simulink model "CONTROLLER_LONG_FG"  (R2015a)
settings: Solver=ode45  StartTime=0.0  StopTime=196  RelTol=1e-3
values from neighbouring files (symbols this model uses):
  A = [-0.0089 -0.1474 0 -9.75; -0.0216 -0.3601 5.9470 -0.151; 0 -0.00015 -0.0224 0.0006; 0 0 1 0]    [controller_design.m]
  B = [-2.682 9.748; 29 3.77; -3.847 -0.034; 0 0]    [controller_design.m]
  C = diag([1 1 1 1])    [controller_design.m]
  D = zeros(4,2)    [controller_design.m]
  K = place(A,B,p)    [controller_design.m]
  tht_tr = 6.30*(pi/180)    (= 0.109955742876)    [controller_design.m]
  u_tr = 155    [controller_design.m]
  w_tr = 0    [controller_design.m]
  XE_0 = 0    [constants.m]    (also in controller_design.m)
  ZE_0 = -2000    [constants.m]    (also in controller_design.m)
undefined symbols (not defined in the file or in its folder): Earth, magnitude, WGS84
libraries: simulink x3, aerolibtransform2 x2, aerolibfltsims x1
settings Model: Creator=vinay  LastModifiedBy=vinay

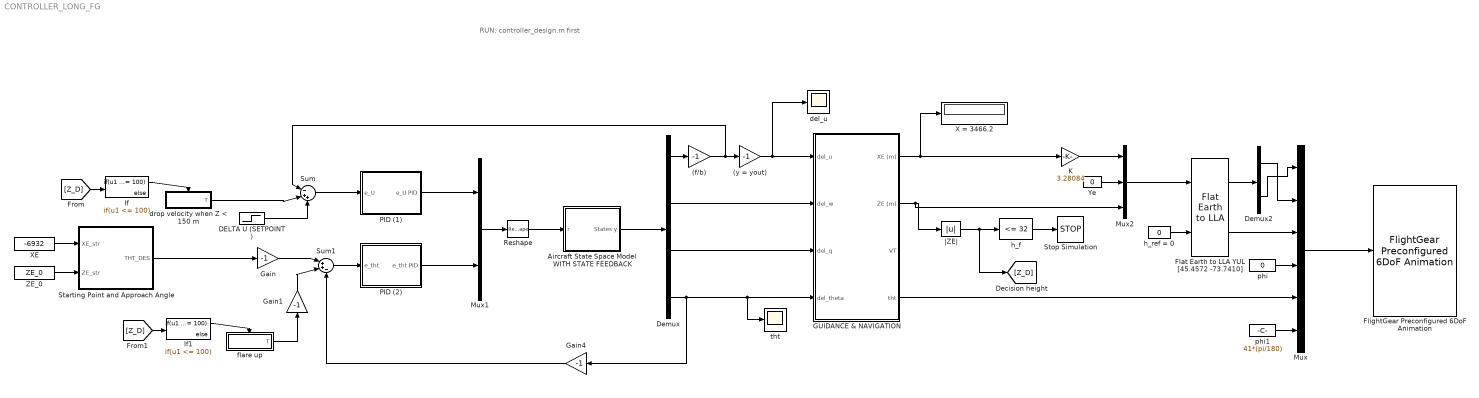
== system CONTROLLER_LONG_FG ==
  note: RUN: controller_design.m first
  (f/b) : Gain  Gain=-1
  (y = yout) : Gain  Gain=-1
  Aircraft State Space Model WITH STATE FEEDBACK : Subsystem
  DELTA U (SETPOINT) : Step  After=36  SampleTime=0
  Demux : Demux
  Demux2 : Demux  Outputs=2
  "Flat Earth to LLA YUL [45.4572 -73.7410] " : aerolibtransform2/Flat Earth to LLA  units=Metric (MKS)  ptype=Earth (WGS84)  F=1/298.257223563  R=6378137  LL0=[45.3027633 -73.9311585]  psi=41
  FlightGear Preconfigured 6DoF Animation : aerolibfltsims/FlightGear Preconfigured 6DoF Animation  xFlightGearVersion=v3.0  DestinationIpAddress=127.0.0.1  DestinationPort=5502  SampleTime=1/30
  "GUIDANCE & NAVIGATION " : Subsystem
  Gain : Gain  Gain=-1
  Gain1 : Gain  Gain=-1
  Gain4 : Gain  Gain=-1
  If : If  IfExpression=u1 <= 100
  If1 : If  IfExpression=u1 <= 100
  K : Gain  Gain=3.28084
  Mux : Mux  Inputs=6
  Mux1 : Mux  Inputs=2
  Mux2 : Mux  Inputs=3
  PID (1) : Subsystem
  PID (2) : Subsystem
  Reshape : Reshape  OutputDimensionality=Customize  OutputDimensions=[2,1]
  Starting Point and Approach Angle : Subsystem
  Stop Simulation : Stop
  Sum : Sum  Inputs=|-++
  Sum1 : Sum  Inputs=|++-
  X = 3466.2 : Display
  "XE " : Constant  Value=-6932
  Ye : Constant  Value=0
  ZE_0 : Constant  Value=ZE_0
  del_u : Scope
      settings: YMin=-1.225e+06  YMax=-800000
  drop velocity when Z < 150 m : Subsystem  TreatAsAtomicUnit=on
  flare up : Subsystem  TreatAsAtomicUnit=on
  h_f : simulink/Logic and Bit Operations/Compare To Constant  relop=<=  const=32  OutDataTypeStr=boolean
  h_ref = 0 : Constant  Value=0
  phi : Constant  Value=0
  phi1 : Constant  Value=41*(pi/180)
  tht : Scope
      settings: YMin=-57500  YMax=-10000
  |ZE| : Abs
  wires:
  Mux1/1 -> Reshape/1
  Reshape/1 -> Aircraft State Space Model WITH STATE FEEDBACK/1(r)
  Aircraft State Space Model WITH STATE FEEDBACK/1(States y) -> Demux/1
  ? -> ?
  Demux/1 -> (f/b)/1
  Gain/1 -> Sum1/1
  Demux/4 -> "GUIDANCE & NAVIGATION "/4(del_theta), tht/1, Gain4/1
  Sum/1 -> PID (1)/1(e_U)
  PID (1)/1(e_U PID) -> Mux1/1
  Sum1/1 -> PID (2)/1(e_tht)
  PID (2)/1(e_tht PID) -> Mux1/2
  Demux/2 -> "GUIDANCE & NAVIGATION "/2(del_w)
  Demux/3 -> "GUIDANCE & NAVIGATION "/3(del_q)
  "GUIDANCE & NAVIGATION "/2(ZE (m)) -> Mux2/3, |ZE|/1
  |ZE|/1 -> [Z_D], h_f/1
  "XE "/1 -> Starting Point and Approach Angle/1(XE_str)
  ZE_0/1 -> Starting Point and Approach Angle/2(ZE_str)
  Starting Point and Approach Angle/1(THT_DES) -> Gain/1
  h_f/1 -> Stop Simulation/1
  (y = yout)/1 -> del_u/1, "GUIDANCE & NAVIGATION "/1(del_u)
  Mux/1 -> FlightGear Preconfigured 6DoF Animation/1
  phi/1 -> Mux/4
  phi1/1 -> Mux/6
  "GUIDANCE & NAVIGATION "/1(XE (m)) -> X = 3466.2/1, K/1
  Ye/1 -> Mux2/2
  Mux2/1 -> "Flat Earth to LLA YUL [45.4572 -73.7410] "/1
  h_ref = 0/1 -> "Flat Earth to LLA YUL [45.4572 -73.7410] "/2
  "Flat Earth to LLA YUL [45.4572 -73.7410] "/1 -> Demux2/1
  "Flat Earth to LLA YUL [45.4572 -73.7410] "/2 -> Mux/3
  Demux2/1 -> Mux/2
  Demux2/2 -> Mux/1
  "GUIDANCE & NAVIGATION "/4(tht) -> Mux/5
  K/1 -> Mux2/1
  DELTA U (SETPOINT)/1 -> Sum/3
  If/1 -> drop velocity when Z < 150 m/Action
  [Z_D] -> If/1
  Gain4/1 -> Sum1/3
  If1/1 -> flare up/Action
  [Z_D] -> If1/1
  drop velocity when Z < 150 m/1(T) -> Sum/2
  (f/b)/1 -> Sum/1, (y = yout)/1
  flare up/1(T) -> Gain1/1
  Gain1/1 -> Sum1/2

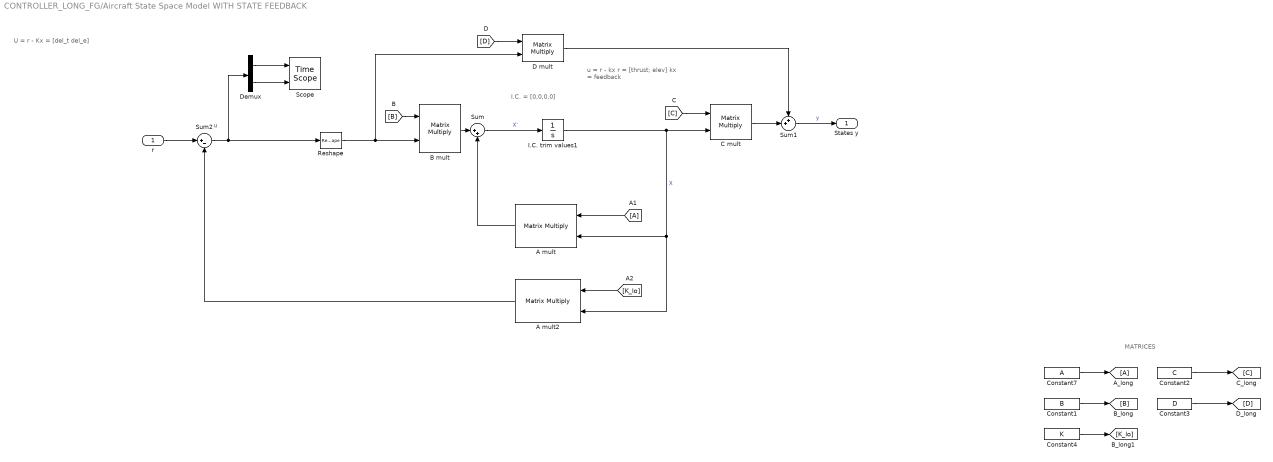
== system CONTROLLER_LONG_FG/Aircraft State Space Model WITH STATE FEEDBACK ==
  note: u
  note: U = r - Kx = [del_t del_e]
  note: u = r - kx
      | r = [thrust; elev]
      | kx = feedback
  note: MATRICES
  note: I.C. = [0,0,0,0]
  r : Inport
  A mult : Product  Multiplication=Matrix(*)  RndMeth=Zero
  A mult2 : Product  Multiplication=Matrix(*)  RndMeth=Zero
  B mult : Product  Multiplication=Matrix(*)  RndMeth=Zero
  C mult : Product  Multiplication=Matrix(*)  RndMeth=Zero
  Constant1 : Constant  Value=B
  Constant2 : Constant  Value=C
  Constant3 : Constant  Value=D
  Constant4 : Constant  Value=K
  Constant7 : Constant  Value=A
  D mult : Product  Multiplication=Matrix(*)  RndMeth=Zero
  Demux : Demux  Outputs=2
  I.C. trim values1 : Integrator  InitialCondition=[0;0;0;0]
  Reshape : Reshape  OutputDimensionality=Customize  OutputDimensions=[2,1]
  Scope : TimeScope  NumInputPorts=2
  Sum : Sum  Inputs=|++
  Sum1 : Sum  Inputs=++|
  Sum2 : Sum  Inputs=|+-
  States y : Outport
  wires:
  Sum/1 -> I.C. trim values1/1  "X'"
  D mult/1 -> Sum1/1
  A mult/1 -> Sum/2
  [B] -> B mult/1
  [A] -> A mult/1
  [D] -> D mult/1
  [C] -> C mult/1
  Sum1/1 -> States y/1  "y"
  B mult/1 -> Sum/1
  C mult/1 -> Sum1/2
  Constant7/1 -> [A]
  Constant1/1 -> [B]
  Constant2/1 -> [C]
  Constant3/1 -> [D]
  Constant4/1 -> [K_lo]
  [K_lo] -> A mult2/1
  A mult2/1 -> Sum2/2
  r/1 -> Sum2/1
  Reshape/1 -> D mult/2, B mult/2
  I.C. trim values1/1 -> C mult/2, A mult2/2, A mult/2  "X"
  Sum2/1 -> Demux/1, Reshape/1
  Demux/1 -> Scope/1
  Demux/2 -> Scope/2

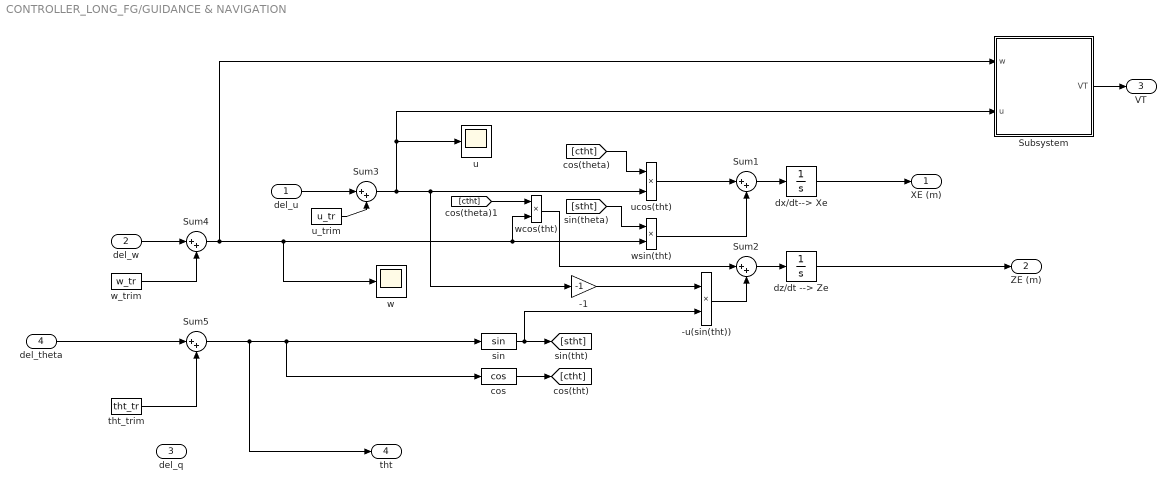
== system CONTROLLER_LONG_FG/GUIDANCE & NAVIGATION  ==
  del_u : Inport
  del_w : Inport  Port=2
  del_q : Inport  Port=3
  del_theta : Inport  Port=4
  -1 : Gain  Gain=-1
  -u(sin(tht)) : Product
  Subsystem : Subsystem
  Sum{1..5} (5 alike) : Sum  Inputs=|++
  cos : Trigonometry  Operator=cos
  dx/dt--> Xe : Integrator  InitialCondition=XE_0
  dz/dt --> Ze : Integrator  InitialCondition=ZE_0
  sin : Trigonometry
  tht_trim : Constant  Value=tht_tr
  u : Scope
      settings: SaveName=ScopeData4
  u_trim : Constant  Value=u_tr
  ucos(tht) : Product
  w : Scope
      settings: SaveName=ScopeData5
  w_trim : Constant  Value=w_tr
  wcos(tht) : Product
  wsin(tht) : Product
  XE (m) : Outport
  ZE (m) : Outport  Port=2
  VT : Outport  Port=3
  tht : Outport  Port=4
  wires:
  [stht] -> wsin(tht)/1
  wsin(tht)/1 -> Sum1/2
  dx/dt--> Xe/1 -> XE (m)/1
  ucos(tht)/1 -> Sum1/1
  dz/dt --> Ze/1 -> ZE (m)/1
  Sum1/1 -> dx/dt--> Xe/1
  Sum2/1 -> dz/dt --> Ze/1
  cos/1 -> [ctht]
  sin/1 -> -u(sin(tht))/2, [stht]
  wcos(tht)/1 -> Sum2/1
  [ctht] -> wcos(tht)/1
  -1/1 -> -u(sin(tht))/1
  [ctht] -> ucos(tht)/1
  -u(sin(tht))/1 -> Sum2/2
  tht_trim/1 -> Sum5/2
  del_u/1 -> Sum3/1
  Sum3/1 -> u/1, Subsystem/2(u), -1/1, ucos(tht)/2
  u_trim/1 -> Sum3/2
  del_w/1 -> Sum4/1
  Sum4/1 -> w/1, wcos(tht)/2, wsin(tht)/2, Subsystem/1(w)
  w_trim/1 -> Sum4/2
  del_theta/1 -> Sum5/1
  Sum5/1 -> tht/1, cos/1, sin/1
  Subsystem/1(VT) -> VT/1

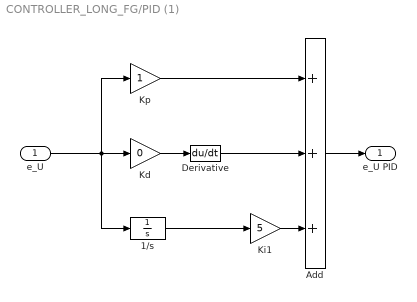
== system CONTROLLER_LONG_FG/PID (1) ==
  e_U : Inport
  1/s : Integrator
  Add : Sum  Inputs=+++
  Derivative : Derivative
  Kd : Gain  Gain=0
  Ki1 : Gain  Gain=5
  Kp : Gain
  e_U PID : Outport
  wires:
  Add/1 -> e_U PID/1
  Kp/1 -> Add/1
  Ki1/1 -> Add/3
  e_U/1 -> 1/s/1, Kd/1, Kp/1
  Kd/1 -> Derivative/1
  Derivative/1 -> Add/2
  1/s/1 -> Ki1/1

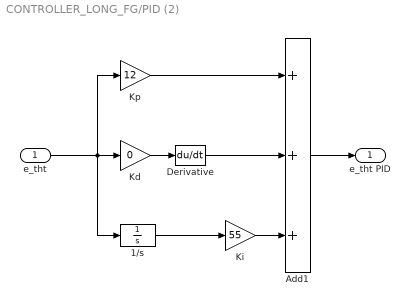
== system CONTROLLER_LONG_FG/PID (2) ==
  e_tht : Inport
  1/s : Integrator
  Add1 : Sum  Inputs=+++
  Derivative : Derivative
  "Kd " : Gain  Gain=0
  "Ki " : Gain  Gain=55
  Kp : Gain  Gain=12
  e_tht PID : Outport
  wires:
  Add1/1 -> e_tht PID/1
  Kp/1 -> Add1/1
  e_tht/1 -> Kp/1, 1/s/1, "Kd "/1
  "Ki "/1 -> Add1/3
  "Kd "/1 -> Derivative/1
  Derivative/1 -> Add1/2
  1/s/1 -> "Ki "/1

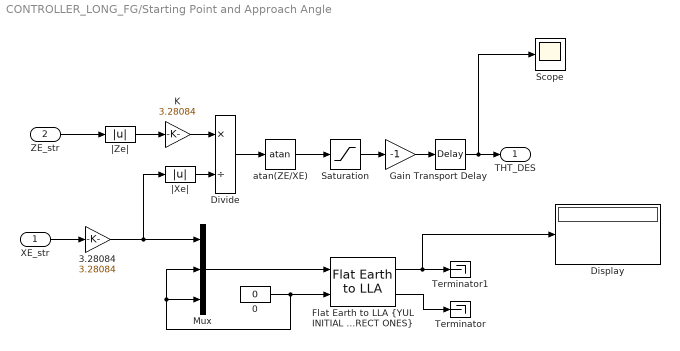
== system CONTROLLER_LONG_FG/Starting Point and Approach Angle ==
  XE_str : Inport
  ZE_str : Inport  Port=2
  0 : Constant  Value=0
  3.28084 : Gain  Gain=3.28084
  Display : Display
  Divide : Product  Inputs=*/
  "Flat Earth to LLA {YUL INITIAL COORDS UPDATED - CORRECT ONES}" : aerolibtransform2/Flat Earth to LLA  units=Metric (MKS)  ptype=Earth (WGS84)  F=1/298.257223563  R=6378137  LL0=[45.4572 -73.7410]  psi=41
  Gain : Gain  Gain=-1
  K : Gain  Gain=3.28084
  Mux : Mux  Inputs=3
  Saturation : Saturate  UpperLimit=0.5235  LowerLimit=-0.5235
  Scope : Scope
      settings: SaveName=ScopeData2
  Terminator : Terminator
  Terminator1 : Terminator
  Transport Delay : TransportDelay
  atan(ZE/XE) : Trigonometry  Operator=atan
  |Xe| : Abs
  |Ze| : Abs
  THT_DES : Outport
  wires:
  Mux/1 -> "Flat Earth to LLA {YUL INITIAL COORDS UPDATED - CORRECT ONES}"/1
  XE_str/1 -> 3.28084/1
  0/1 -> Mux/2, Mux/3, "Flat Earth to LLA {YUL INITIAL COORDS UPDATED - CORRECT ONES}"/2
  ZE_str/1 -> |Ze|/1
  |Ze|/1 -> K/1
  |Xe|/1 -> Divide/2
  Divide/1 -> atan(ZE/XE)/1
  "Flat Earth to LLA {YUL INITIAL COORDS UPDATED - CORRECT ONES}"/2 -> Terminator/1
  Saturation/1 -> Gain/1
  atan(ZE/XE)/1 -> Saturation/1
  Gain/1 -> Transport Delay/1
  Transport Delay/1 -> Scope/1, THT_DES/1
  "Flat Earth to LLA {YUL INITIAL COORDS UPDATED - CORRECT ONES}"/1 -> Display/1, Terminator1/1
  3.28084/1 -> |Xe|/1, Mux/1
  K/1 -> Divide/1

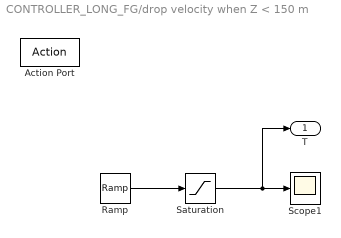
== system CONTROLLER_LONG_FG/drop velocity when Z < 150 m ==
  Action Port : ActionPort  ActionType=then
  Ramp : simulink/Sources/Ramp  slope=5  start=0  X0=0
  Saturation : Saturate  UpperLimit=15  LowerLimit=0
  Scope1 : Scope
      settings: TimeRange=11  YMin=0  YMax=3.5  SaveName=ScopeData2
  T : Outport
  wires:
  Ramp/1 -> Saturation/1
  Saturation/1 -> T/1, Scope1/1

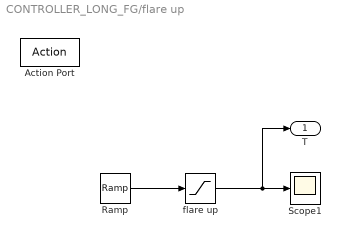
== system CONTROLLER_LONG_FG/flare up ==
  Action Port : ActionPort  ActionType=then
  Ramp : simulink/Sources/Ramp  slope=0.35  start=0  X0=0
  Scope1 : Scope
      settings: TimeRange=11  YMin=0  YMax=3.5  SaveName=ScopeData2
  flare up : Saturate  UpperLimit=0.7403  LowerLimit=0
  T : Outport
  wires:
  Ramp/1 -> flare up/1
  flare up/1 -> T/1, Scope1/1

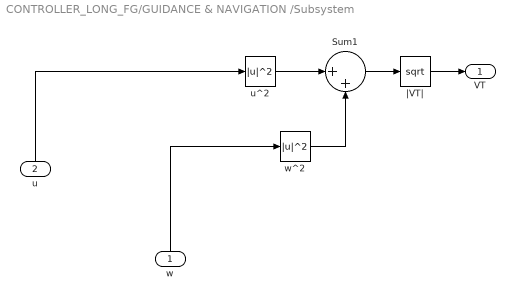
== system CONTROLLER_LONG_FG/GUIDANCE & NAVIGATION /Subsystem ==
  w : Inport
  u : Inport  Port=2
  Sum1 : Sum  Inputs=|++
  u^2 : Math  Operator=magnitude^2  SaturateOnIntegerOverflow=on
  w^2 : Math  Operator=magnitude^2  SaturateOnIntegerOverflow=on
  |VT| : Sqrt  SaturateOnIntegerOverflow=on
  VT : Outport
  wires:
  Sum1/1 -> |VT|/1
  |VT|/1 -> VT/1
  u^2/1 -> Sum1/1
  w^2/1 -> Sum1/2
  w/1 -> w^2/1
  u/1 -> u^2/1
